simulink model "spring_mass_damp"  (R2021a)
settings: Solver=VariableStepAuto  StartTime=0.0  StopTime=1000  RelTol=1e-3
values from neighbouring files (symbols this model uses):
  c = 0.5    [spring_og_sys.m]    (also in spring_og_sys_id.m; spring_tf.mat)
  k = 400    [generate_data.m]    (also in spring_og_sys.m = 0.8; spring_og_sys_id.m = 0.8; spring_sys_id.m = 300; spring_tf.mat = 0.8)
  m = 10    [generate_data.m]    (also in spring_og_sys.m; spring_og_sys_id.m; spring_sys_id.m = 5; spring_tf.mat)
libraries: simulink x1
settings Model: Creator=probinet  LastModifiedBy=probinet

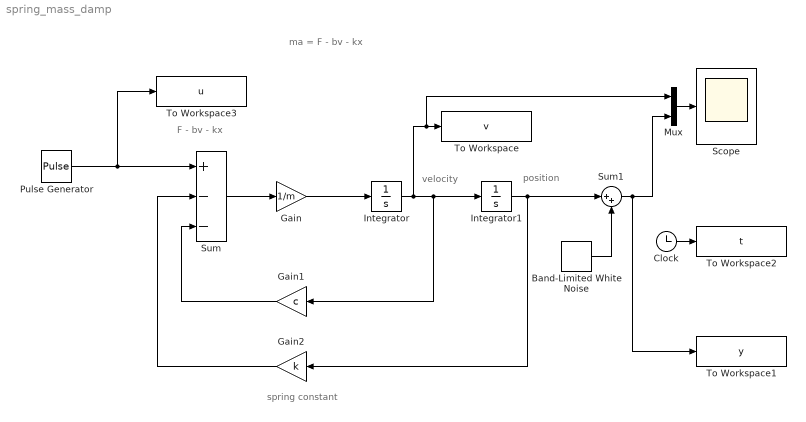
== system spring_mass_damp ==
  note: spring constant
  note: ma = F - bv - kx
  note: F - bv - kx
  note: velocity
  note: position
  Band-Limited White Noise : simulink/Sources/Band-Limited White Noise  Cov=n  Ts=0.1  seed=[23341]
  Clock : Clock
  Gain : Gain  Gain=1/m
  Gain1 : Gain  Gain=c
  Gain2 : Gain  Gain=k
  Integrator : Integrator
  Integrator1 : Integrator
  Mux : Mux  Inputs=2
  Pulse Generator : DiscretePulseGenerator  PulseType=Time based  Period=500  PulseWidth=50
  Scope : Scope
  Sum : Sum  Inputs=+--
  Sum1 : Sum  Inputs=|++
  To Workspace : ToWorkspace  VariableName=v  SampleTime=-1
      settings: Save2DSignal=2-D array (concatenate along first dimension)
  To Workspace1 : ToWorkspace  VariableName=y  SampleTime=-1
      settings: Save2DSignal=2-D array (concatenate along first dimension)
  To Workspace2 : ToWorkspace  VariableName=t  SampleTime=-1
      settings: Save2DSignal=2-D array (concatenate along first dimension)
  To Workspace3 : ToWorkspace  VariableName=u  SampleTime=-1
      settings: Save2DSignal=2-D array (concatenate along first dimension)
  wires:
  Gain/1 -> Integrator/1
  Integrator/1 -> Integrator1/1, Gain1/1, Mux/1, To Workspace/1
  Integrator1/1 -> Sum1/1, Gain2/1
  Gain1/1 -> Sum/3
  Gain2/1 -> Sum/2
  Sum/1 -> Gain/1
  Pulse Generator/1 -> To Workspace3/1, Sum/1
  Clock/1 -> To Workspace2/1
  Band-Limited White Noise/1 -> Sum1/2
  Sum1/1 -> To Workspace1/1, Mux/2
  Mux/1 -> Scope/1
